simulink model "different_inverter_controls_BPS"  (R2024b)
settings: Solver=ode4  StartTime=0.0  StopTime=5  FixedStep=Ts  RelTol=1e-3
InitFcn:
  | %mode_of_operation=1;
  | %BESS_control_mode=1;
  | %Gen_Q_Control =1;
  | 
  | %Exciter_init;
  | 
  | %Exciter_init
  | Xq=0.474;
  | %%====================================================
  | % ST6C Exciter Parameters
  | 
  | KPA=30;
  | KIA=59.91;
  | KFF=1;
  | KM=1;
  | KLR=22.47;
  | KCL=1.04;
  | VAMAX=7.05;
  | VAMIN=-6.11;
  | VRMAX=7.05;
  | VRMIN=-6.11;
  | ILR=5.02;
  | KG=1;
  | TG=0.024;
  | TA=0.01;
  | VBMAX=999;
  | VMMAX=7.05;
  | VMMIN=-6.11;
  | KI=0;
  | Kp=1;
  | Kc=0;
  | Vt0=0;
  | VAAMAX=VAMAX;
  | %%========================================================
  | % UEL2C parameters
  | 
  | TUQ=.005;
  | TUP=0.050;
  | TUV=0.2;
  | TQREF=0;
  | Tadj=0;
  | K1=0;
  | K2=2;
  | VBIAS=1;
  | KFB=0;
  | TUL=0;
  | VUImax=1;
  | VUImin=-1;
  | VUELmax1=1;
  | VUELmax2=1;
  | VUELmin1=-1;
  | VUELmin2=-1;
  | KUF=0;
  | KUL=0.24;
  | KUI=0.001;
  | TU1=0;TU2=0;TU3=0;TU4=0;
  | KFIX=1;
  | VF=0;
  | VFB=0;
  | %%===========================================================
  | ... (+60 lines)
values from neighbouring files (symbols this model uses):
  inv1 = struct    [multiInverterParams.m]
  kp_sync = KQ_p/10    (= 0.04)    [multiInverterParams.m]
  Vdc = 1000    [multiInverterParams.m]
  Vpp = 480    [multiInverterParams.m]
undefined symbols (not defined in the file or in its folder): D1, Delta, DiscIntNeverNeededParam, Ion, Lithium, sigbuilder_block, sps
libraries: slpidlib x34, spsThreePhaseVIMeasurementLib x31, spsThreePhaseSeriesRLCBranchLib x23, spsabctodq0Lib x22, spsPower3phInstantaneousLib x22, spsThreePhaseTransformerTwoWindingsLib x16, spsSeriesRLCBranchLib x16, spsThreePhaseSeriesRLCLoadLib x14, simulink x12, spsPLL3phLib x11, spsGroundLib x9, powerlib_extras x8
(part 8 of 9)

== system different_inverter_controls_BPS/IBR-GFM PV Droop/IBR/Power Controller/P,Q Control /Integrator1 ==
  w : Inport
  Constant1 : Constant  Commented=on  Value=2*pi  SampleTime=Ts
  Constant2 : Constant  Value=2*pi  SampleTime=Ts_Control
  Constant3 : Constant  Commented=on  Value=2*pi  SampleTime=Ts
  Constant4 : Constant  Commented=on  Value=f  SampleTime=Ts_Control
  Constant5 : Constant  Commented=on  Value=0  SampleTime=Ts_Control
  Discrete-Time Integrator : DiscreteIntegrator  Commented=on  IntegratorMethod=Integration: Trapezoidal  SampleTime=Ts  ICPrevOutput=DiscIntNeverNeededParam  ICPrevScaledInput=DiscIntNeverNeededParam
  Discrete-Time Integrator1 : DiscreteIntegrator  ExternalReset=rising  InitialConditionSource=external  SampleTime=Ts_Control  ShowStatePort=on  ICPrevOutput=DiscIntNeverNeededParam  ICPrevScaledInput=DiscIntNeverNeededParam
  Divide : Product  Commented=on  Inputs=*/
  From : From  Commented=on  GotoTag=fsys
  Gain : Gain  Commented=on  Gain=2*pi*f
  Gain1 : Gain  Commented=on  Gain=2*pi*f  SaturateOnIntegerOverflow=on  OutDataTypeStr=Inherit: Same as input  ParamDataTypeStr=Inherit: Same as input
  Gain3 : Gain  Gain=2*pi*f
  Hit Crossing : HitCross  Commented=on  HitCrossingOffset=pi  HitCrossingDirection=falling  ShowOutputPort=off
  Initial : InitialCondition  Value=0
  Initial1 : InitialCondition  Commented=on  Value=0
  Integrator : Integrator  Commented=on  ExternalReset=rising  InitialConditionSource=external  InitialCondition=sps.Phase_Init*pi/180  LimitOutput=on  ShowStatePort=on
  Integrator2 : Integrator  Commented=on  ExternalReset=rising  InitialConditionSource=external  InitialCondition=sps.Phase_Init*pi/180  ShowStatePort=on
  Math Function : Math  Commented=on  Operator=mod  SignedPower=on
  Relational Operator : RelationalOperator  Operator=>  OutDataTypeStr=boolean  InputSameDT=off
  Relational Operator1 : RelationalOperator  Commented=on  Operator=>  OutDataTypeStr=boolean  InputSameDT=off
  Scope : Scope
  Scope1 : Scope  Commented=on
  Scope2 : Scope  Commented=on
  Scope3 : Scope  Commented=on
  Subtract : Sum  Inputs=+-
  Subtract1 : Sum  Commented=on  Inputs=+-
  Sum1 : Sum  Commented=on  Inputs=|++
  Sum2 : Sum  Commented=on  Inputs=|+-
  Theta : Outport
  wires:
  Gain3/1 -> Discrete-Time Integrator1/1
  w/1 -> Sum2/1, Gain3/1
  Gain1/1 -> Integrator/1
  Initial1/1 -> Integrator/3
  Relational Operator1/1 -> Integrator/2
  Integrator/State -> Subtract1/1, Relational Operator1/1
  Constant1/1 -> Subtract1/2, Relational Operator1/2
  Integrator/1 -> Scope3/1, Hit Crossing/1
  Subtract1/1 -> Initial1/1
  Relational Operator/1 -> Discrete-Time Integrator1/2
  Initial/1 -> Discrete-Time Integrator1/3
  Discrete-Time Integrator1/State -> Subtract/1, Relational Operator/1
  Constant2/1 -> Subtract/2, Relational Operator/2
  Subtract/1 -> Initial/1
  Discrete-Time Integrator1/1 -> Scope/1, Theta/1
  Gain/1 -> Discrete-Time Integrator/1
  Discrete-Time Integrator/1 -> Math Function/1
  Constant3/1 -> Math Function/2
  Math Function/1 -> Scope1/1
  Sum1/1 -> Gain/1  "W"
  Constant5/1 -> Sum2/2
  Sum2/1 -> Scope2/1, Sum1/1  "W"
  From/1 -> Divide/1
  Constant4/1 -> Divide/2
  Divide/1 -> Sum1/2

== system different_inverter_controls_BPS/IBR-GFM Synchro-inverter/Inverter/Inverter Control/Current Control/Current Regulator ==
  note: Id positive --> The converter generates active power ("Inverter mode") = Active Power P positive
  note: Iq positive --> The converter absorbs reactive power ("Inductive mode") = Reactive Power Q negative
  note: Sign Convention: Current going out of the converter = positive current
  note: Current Regulator
      | ================
  VdVq_meas : Inport  PortDimensions=2
  IdIq_meas : Inport  Port=2  PortDimensions=2
  IdIq_ref : Inport  Port=3  PortDimensions=2
  Add1 : Sum  Inputs=++-
  Add2 : Sum
  Add3 : Sum  Inputs=+++
  Demux : Demux  Outputs=2
  Demux1 : Demux  Outputs=2
  Lff : Gain  Gain=inv1.Lpu  SaturateOnIntegerOverflow=on  OutDataTypeStr=Inherit: Same as input  ParamDataTypeStr=Inherit: Same as input
  "Lff  " : Gain  Gain=inv1.Lpu  SaturateOnIntegerOverflow=on  OutDataTypeStr=Inherit: Same as input  ParamDataTypeStr=Inherit: Same as input
  Lff  1 : Gain  Commented=on  Gain=Ltot_pu  SaturateOnIntegerOverflow=on  OutDataTypeStr=Inherit: Same as input  ParamDataTypeStr=Inherit: Same as input
  Mux : Mux  Inputs=2
  PI : slpidlib/PID Controller  Controller=PI  Form=Parallel  TimeDomain=Discrete-time  UseExternalTs=off  SampleTime=Ts_Control  IntegratorMethod=Forward Euler  FilterMethod=Forward Euler  ControllerParametersSource=internal  P=Kp_Ireg/10  I=Ki_Ireg  D=0  UseFilter=on  N=100  TunerSelectOption=Transfer Function Based (PID Tuner App)  InitialConditionSource=internal  InitialConditionForIntegrator=0  InitialConditionForFilter=0  DifferentiatorICPrevScaledInput=0  ExternalReset=none  TrackingMode=off  Kt=1  LimitOutput=on  SatLimitsSource=internal  UpperSaturationLimit=1.5  LowerSaturationLimit=-1.5  LinearizeAsGain=off  AntiWindupMode=back-calculation  Kb=1  POutMin=[]  POutMax=[]  IOutMin=[]  IOutMax=[]  DOutMin=[]  DOutMax=[]  NOutMin=[]  NOutMax=[]  SumOutMin=[]  SumOutMax=[]  SaturationOutMin=[]  SaturationOutMax=[]  PParamMin=[]  PParamMax=[]  IParamMin=[]  IParamMax=[]  DParamMin=[]  DParamMax=[]  NParamMin=[]  NParamMax=[]  KbParamMin=[]  KbParamMax=[]  KtParamMin=[]  KtParamMax=[]  KbOutMin=[]  KbOutMax=[]  KtOutMin=[]  KtOutMax=[]  IntegratorOutMin=[]  IntegratorOutMax=[]  FilterOutMin=[]  FilterOutMax=[]  SumI1OutMin=[]  SumI1OutMax=[]  SumI2OutMin=[]  SumI2OutMax=[]  SumI3OutMin=[]  SumI3OutMax=[]  SumI4OutMin=[]  SumI4OutMax=[]  SumDOutMin=[]  SumDOutMax=[]  DifferentiatorOutMin=[]  DifferentiatorOutMax=[]  FilterDiffOutCoefMin=[]  FilterDiffOutCoefMax=[]  ReciprocalOutMin=[]  ReciprocalOutMax=[]  SumDenOutMin=[]  SumDenOutMax=[]  SumNumOutMin=[]  SumNumOutMax=[]  DivideOutMin=[]  DivideOutMax=[]  UdiffTsProdOutMin=[]  UdiffTsProdOutMax=[]  NTsProdOutMin=[]  NTsProdOutMax=[]  UintegralTsProdOutMin=[]  UintegralTsProdOutMax=[]  UngainTsProdOutMin=[]  UngainTsProdOutMax=[]  FilterDenConstantOutDataTypeStr=Inherit: Inherit via back propagation  FilterDenConstantOutMin=[]  FilterDenConstantOutMax=[]  PCopyOutDataTypeStr=Inherit: Inherit via back propagation  PCopyOutMin=[]  PCopyOutMax=[]  NCopyOutDataTypeStr=Inherit: Inherit via back propagation  NCopyOutMin=[]  NCopyOutMax=[]  IntegratorContinuousStateAttributes=''  IntegratorStateMustResolveToSignalObject=off  IntegratorRTWStateStorageClass=Auto  FilterContinuousStateAttributes=''  FilterStateMustResolveToSignalObject=off  FilterRTWStateStorageClass=Auto  ParallelPVariant=InternalParameters  IdealPVariant=Disabled  IVariant=InternalParameters  DVariant=Disabled  IntegratorVariant=Discrete  SatVariant=Enabled  AWVariant=BackCalculation  PCopyVariant=Disabled  TRVariant=Disabled  FdbkBlocksVariant=Forward  IdealPFdbkVariant=Disabled  SatFdbkVariant=Disabled  DerivativeFilterVariant=Disabled  NVariant=Disabled  NCopyVariant=Disabled_SignalSpec  FilterICVariant=Disabled  IntegratorICVariant=InternalICs  ExternalResetVariant=Disabled  TRSumVariant=Passthrough  SumFdbkVariant=Disabled  SumVariant=Sum_PI  TsampFilterVariant=InternalTs  TsampNgainVariant=Passthrough  TsampIntegralVariant=Passthrough  ExternalSaturationOutDataTypeStr=Inherit: Same as second input
  PI1 : slpidlib/PID Controller  Commented=on  Controller=PI  Form=Parallel  TimeDomain=Discrete-time  UseExternalTs=off  SampleTime=Ts_Control  IntegratorMethod=Forward Euler  FilterMethod=Forward Euler  ControllerParametersSource=internal  P=Kp_Ireg  I=Ki_Ireg  D=0  UseFilter=on  N=100  TunerSelectOption=Transfer Function Based (PID Tuner App)  InitialConditionSource=internal  InitialConditionForIntegrator=0  InitialConditionForFilter=0  DifferentiatorICPrevScaledInput=0  ExternalReset=none  TrackingMode=off  Kt=1  LimitOutput=on  SatLimitsSource=internal  UpperSaturationLimit=1.5  LowerSaturationLimit=-1.5  LinearizeAsGain=off  AntiWindupMode=clamping  Kb=1  POutMin=[]  POutMax=[]  IOutMin=[]  IOutMax=[]  DOutMin=[]  DOutMax=[]  NOutMin=[]  NOutMax=[]  SumOutMin=[]  SumOutMax=[]  SaturationOutMin=[]  SaturationOutMax=[]  PParamMin=[]  PParamMax=[]  IParamMin=[]  IParamMax=[]  DParamMin=[]  DParamMax=[]  NParamMin=[]  NParamMax=[]  KbParamMin=[]  KbParamMax=[]  KtParamMin=[]  KtParamMax=[]  KbOutMin=[]  KbOutMax=[]  KtOutMin=[]  KtOutMax=[]  IntegratorOutMin=[]  IntegratorOutMax=[]  FilterOutMin=[]  FilterOutMax=[]  SumI1OutMin=[]  SumI1OutMax=[]  SumI2OutMin=[]  SumI2OutMax=[]  SumI3OutMin=[]  SumI3OutMax=[]  SumI4OutMin=[]  SumI4OutMax=[]  SumDOutMin=[]  SumDOutMax=[]  DifferentiatorOutMin=[]  DifferentiatorOutMax=[]  FilterDiffOutCoefMin=[]  FilterDiffOutCoefMax=[]  ReciprocalOutMin=[]  ReciprocalOutMax=[]  SumDenOutMin=[]  SumDenOutMax=[]  SumNumOutMin=[]  SumNumOutMax=[]  DivideOutMin=[]  DivideOutMax=[]  UdiffTsProdOutMin=[]  UdiffTsProdOutMax=[]  NTsProdOutMin=[]  NTsProdOutMax=[]  UintegralTsProdOutMin=[]  UintegralTsProdOutMax=[]  UngainTsProdOutMin=[]  UngainTsProdOutMax=[]  FilterDenConstantOutDataTypeStr=Inherit: Inherit via back propagation  FilterDenConstantOutMin=[]  FilterDenConstantOutMax=[]  PCopyOutDataTypeStr=Inherit: Inherit via back propagation  PCopyOutMin=[]  PCopyOutMax=[]  NCopyOutDataTypeStr=Inherit: Inherit via back propagation  NCopyOutMin=[]  NCopyOutMax=[]  IntegratorContinuousStateAttributes=''  IntegratorStateMustResolveToSignalObject=off  IntegratorRTWStateStorageClass=Auto  FilterContinuousStateAttributes=''  FilterStateMustResolveToSignalObject=off  FilterRTWStateStorageClass=Auto  ParallelPVariant=InternalParameters  IdealPVariant=Disabled  IVariant=InternalParameters  DVariant=Disabled  IntegratorVariant=Discrete  SatVariant=Enabled  AWVariant=DiscClampingParallel  PCopyVariant=Disabled  TRVariant=Disabled  FdbkBlocksVariant=Forward  IdealPFdbkVariant=Disabled  SatFdbkVariant=Disabled  DerivativeFilterVariant=Disabled  NVariant=Disabled  NCopyVariant=Disabled_SignalSpec  FilterICVariant=Disabled  IntegratorICVariant=InternalICs  ExternalResetVariant=Disabled  TRSumVariant=Passthrough  SumFdbkVariant=Disabled  SumVariant=Sum_PI  TsampFilterVariant=InternalTs  TsampNgainVariant=Passthrough  TsampIntegralVariant=Passthrough  ExternalSaturationOutDataTypeStr=Inherit: Same as second input
  PI2 : slpidlib/PID Controller  Commented=on  Controller=PI  Form=Parallel  TimeDomain=Discrete-time  UseExternalTs=off  SampleTime=Ts_Control  IntegratorMethod=Forward Euler  FilterMethod=Forward Euler  ControllerParametersSource=internal  P=Kp_Ireg  I=Ki_Ireg  D=0  UseFilter=on  N=100  TunerSelectOption=Transfer Function Based (PID Tuner App)  InitialConditionSource=internal  InitialConditionForIntegrator=0  InitialConditionForFilter=0  DifferentiatorICPrevScaledInput=0  ExternalReset=none  TrackingMode=off  Kt=1  LimitOutput=on  SatLimitsSource=internal  UpperSaturationLimit=1.5  LowerSaturationLimit=-1.5  LinearizeAsGain=off  AntiWindupMode=back-calculation  Kb=1  POutMin=[]  POutMax=[]  IOutMin=[]  IOutMax=[]  DOutMin=[]  DOutMax=[]  NOutMin=[]  NOutMax=[]  SumOutMin=[]  SumOutMax=[]  SaturationOutMin=[]  SaturationOutMax=[]  PParamMin=[]  PParamMax=[]  IParamMin=[]  IParamMax=[]  DParamMin=[]  DParamMax=[]  NParamMin=[]  NParamMax=[]  KbParamMin=[]  KbParamMax=[]  KtParamMin=[]  KtParamMax=[]  KbOutMin=[]  KbOutMax=[]  KtOutMin=[]  KtOutMax=[]  IntegratorOutMin=[]  IntegratorOutMax=[]  FilterOutMin=[]  FilterOutMax=[]  SumI1OutMin=[]  SumI1OutMax=[]  SumI2OutMin=[]  SumI2OutMax=[]  SumI3OutMin=[]  SumI3OutMax=[]  SumI4OutMin=[]  SumI4OutMax=[]  SumDOutMin=[]  SumDOutMax=[]  DifferentiatorOutMin=[]  DifferentiatorOutMax=[]  FilterDiffOutCoefMin=[]  FilterDiffOutCoefMax=[]  ReciprocalOutMin=[]  ReciprocalOutMax=[]  SumDenOutMin=[]  SumDenOutMax=[]  SumNumOutMin=[]  SumNumOutMax=[]  DivideOutMin=[]  DivideOutMax=[]  UdiffTsProdOutMin=[]  UdiffTsProdOutMax=[]  NTsProdOutMin=[]  NTsProdOutMax=[]  UintegralTsProdOutMin=[]  UintegralTsProdOutMax=[]  UngainTsProdOutMin=[]  UngainTsProdOutMax=[]  FilterDenConstantOutDataTypeStr=Inherit: Inherit via back propagation  FilterDenConstantOutMin=[]  FilterDenConstantOutMax=[]  PCopyOutDataTypeStr=Inherit: Inherit via back propagation  PCopyOutMin=[]  PCopyOutMax=[]  NCopyOutDataTypeStr=Inherit: Inherit via back propagation  NCopyOutMin=[]  NCopyOutMax=[]  IntegratorContinuousStateAttributes=''  IntegratorStateMustResolveToSignalObject=off  IntegratorRTWStateStorageClass=Auto  FilterContinuousStateAttributes=''  FilterStateMustResolveToSignalObject=off  FilterRTWStateStorageClass=Auto  ParallelPVariant=InternalParameters  IdealPVariant=Disabled  IVariant=InternalParameters  DVariant=Disabled  IntegratorVariant=Discrete  SatVariant=Enabled  AWVariant=BackCalculation  PCopyVariant=Disabled  TRVariant=Disabled  FdbkBlocksVariant=Forward  IdealPFdbkVariant=Disabled  SatFdbkVariant=Disabled  DerivativeFilterVariant=Disabled  NVariant=Disabled  NCopyVariant=Disabled_SignalSpec  FilterICVariant=Disabled  IntegratorICVariant=InternalICs  ExternalResetVariant=Disabled  TRSumVariant=Passthrough  SumFdbkVariant=Disabled  SumVariant=Sum_PI  TsampFilterVariant=InternalTs  TsampNgainVariant=Passthrough  TsampIntegralVariant=Passthrough  ExternalSaturationOutDataTypeStr=Inherit: Same as second input
  Rff : Gain  Commented=on  Gain=inv1.R/inv1.Zb  SaturateOnIntegerOverflow=on  OutDataTypeStr=Inherit: Same as input  ParamDataTypeStr=Inherit: Same as input
  "Rff " : Gain  Commented=on  Gain=inv1.R/inv1.Zb  SaturateOnIntegerOverflow=on  OutDataTypeStr=Inherit: Same as input  ParamDataTypeStr=Inherit: Same as input
  Rff 1 : Gain  Commented=on  Gain=Rtot_pu  SaturateOnIntegerOverflow=on  OutDataTypeStr=Inherit: Same as input  ParamDataTypeStr=Inherit: Same as input
  Saturation : Saturate  UpperLimit=1.5  LowerLimit=-1.5
  Scope : Scope  NumInputPorts=2
  Scope1 : Scope
  Sum : Sum  Inputs=|-+
  VdVq_conv : Outport  VectorParamsAs1DForOutWhenUnconnected=off
  wires:
  Add3/1 -> Mux/2
  Demux/2 -> Add3/1
  Add1/1 -> Mux/1  "Feedforward"
  Lff/1 -> Add3/3
  Rff/1 -> Add3/2
  Demux1/2 -> Rff/1, "Lff  "/1
  "Lff  "/1 -> Add1/3
  Demux1/1 -> Lff/1, "Rff "/1
  "Rff "/1 -> Add1/2
  Demux/1 -> Add1/1
  VdVq_meas/1 -> Demux/1
  Saturation/1 -> VdVq_conv/1, Scope1/1
  Add2/1 -> Saturation/1
  IdIq_meas/1 -> Sum/1, Demux1/1
  IdIq_ref/1 -> Sum/2
  Sum/1 -> PI/1, Scope/1
  PI/1 -> Add2/1, Scope/2  "PI"
  Mux/1 -> Add2/2

== system different_inverter_controls_BPS/IBR-GFM Synchro-inverter/Inverter/Inverter Control/Current Control/Uabc_ref Generation max (m) = 1 ==
  note: Uref Generation
      | ==============
  note: (Correction for delay of Ts_Control)
  note: (Correction for transformer
      |  D1 connection)
  wt : Inport
  VdVq_conv : Inport  Port=2
  Add1 : Sum  Inputs=++++
  Add2 : Sum
  Complex to Magnitude-Angle : ComplexToMagnitudeAngle
  Constant : Constant  Commented=on  Value=-pi/6
  Constant1 : Constant  Commented=on  Value=Vnom_dc
  Constant2 : Constant  Value="[ 0  -2*pi/3  2*pi/3  ]"
  Constant3 : Constant  Commented=on  Value=Vnom_sec*sqrt(2)/sqrt(3)
  Constant4 : Constant  Value=Ts_Control*Fnom*(2*pi)
  Constant5 : Constant  Value=Vdc
  Constant6 : Constant  Value=Vpp*sqrt(2)/sqrt(3)
  Demux1 : Demux  Outputs=2
  Gain1 : Gain  Gain=1/2
  Product : Product  Inputs=*/  RndMeth=Zero
  Product1 : Product  Inputs=*/  RndMeth=Zero
  Product2 : Product  Inputs=**  RndMeth=Zero
  Real-Imag to Complex : RealImagToComplex
  Trigonometric Function : Trigonometry
  Uabc_ref : Outport  VectorParamsAs1DForOutWhenUnconnected=off
  wires:
  Product/1 -> Product1/2
  Constant4/1 -> Add1/4
  wt/1 -> Add1/1
  Product2/1 -> Uabc_ref/1
  Trigonometric Function/1 -> Product2/2
  Complex to Magnitude-Angle/1 -> Product2/1
  Add2/1 -> Trigonometric Function/1
  Add1/1 -> Add2/2
  Complex to Magnitude-Angle/2 -> Add2/1
  Constant6/1 -> Product/2
  Constant/1 -> Add1/3
  Constant2/1 -> Add1/2
  Demux1/2 -> Real-Imag to Complex/2
  Demux1/1 -> Real-Imag to Complex/1
  Real-Imag to Complex/1 -> Complex to Magnitude-Angle/1
  Gain1/1 -> Product/1
  Product1/1 -> Demux1/1
  VdVq_conv/1 -> Product1/1
  Constant5/1 -> Gain1/1

== system different_inverter_controls_BPS/IBR-GFM Synchro-inverter/Inverter/Inverter Control/current limiter/P priority limit ==
  idiqP : Inport
  Demux4 : Demux  Outputs=2
  IqLimit : Subsystem
  Mux4 : Mux  Inputs=2
  Rtot_pu1 : Gain  Gain=-1  SaturateOnIntegerOverflow=on  OutDataTypeStr=Inherit: Same as input  ParamDataTypeStr=Inherit: Same as input
  Saturation : Saturate  UpperLimit=limMax  LowerLimit=0
  Saturation Dynamic : simulink/Discontinuities/Saturation Dynamic  OutMin=[]  OutMax=[limMax]  OutDataTypeStr=Inherit: Same as second input  OutDataType=fixdt(1, 16)  OutScaling=2^-10  DoSatur=off
  idiqPRefL : Outport
  wires:
  Saturation Dynamic/1 -> Mux4/2
  idiqP/1 -> Demux4/1
  Demux4/2 -> Saturation Dynamic/2
  Mux4/1 -> idiqPRefL/1
  Demux4/1 -> Saturation/1
  Saturation/1 -> IqLimit/1(In1), Mux4/1
  Rtot_pu1/1 -> Saturation Dynamic/3
  IqLimit/1(Out2) -> Rtot_pu1/1, Saturation Dynamic/1

== system different_inverter_controls_BPS/IBR-GFM Synchro-inverter/Inverter/Inverter Control/current limiter/Q priority limit ==
  idiqP : Inport
  V_inv_mag : Inport  Port=2
  Demux4 : Demux  Outputs=2
  Iq condition : Switch  Threshold=0.9  SaturateOnIntegerOverflow=off  InputSameDT=off
  IqLimit : Subsystem
  Mux4 : Mux  Inputs=2
  Rtot_pu1 : Gain  Gain=-1  SaturateOnIntegerOverflow=on  OutDataTypeStr=Inherit: Same as input  ParamDataTypeStr=Inherit: Same as input
  Saturation : Saturate  UpperLimit=limMax  LowerLimit=limMin
  Saturation Dynamic : simulink/Discontinuities/Saturation Dynamic  OutMin=[]  OutMax=[]  OutDataTypeStr=Inherit: Same as second input  OutDataType=fixdt(1, 16)  OutScaling=2^-10  DoSatur=off
  Saturation1 : Saturate  UpperLimit=0  LowerLimit=limMin
  Scope : Scope
  idiqPRefL : Outport
  wires:
  Iq condition/1 -> Mux4/2, IqLimit/1(In1)
  V_inv_mag/1 -> Iq condition/2
  Saturation/1 -> Iq condition/1
  idiqP/1 -> Demux4/1
  Mux4/1 -> idiqPRefL/1
  Rtot_pu1/1 -> Saturation Dynamic/3
  Saturation Dynamic/1 -> Mux4/1
  Demux4/1 -> Saturation Dynamic/2
  IqLimit/1(Out2) -> Rtot_pu1/1, Saturation Dynamic/1
  Saturation1/1 -> Iq condition/3
  Demux4/2 -> Saturation/1, Saturation1/1

== system different_inverter_controls_BPS/IBR-GFM Synchro-inverter/Inverter/Inverter Control/current limiter/Subsystem3 ==
  In1 : Inport
  Demux2 : Demux  Outputs=2
  Math Function : Math  Operator=square  SignedPower=on
  Saturation : Saturate  UpperLimit=limMax  LowerLimit=limMin
  Scope : Scope  NumInputPorts=2
  Sqrt1 : Sqrt
  Subtract : Sum
  Out1 : Outport
  Out2 : Outport  Port=2
  wires:
  Demux2/2 -> Subtract/2
  Demux2/1 -> Subtract/1
  Math Function/1 -> Demux2/1
  In1/1 -> Scope/2, Math Function/1
  Subtract/1 -> Sqrt1/1  "Ipos2"
  Sqrt1/1 -> Saturation/1, Scope/1, Out2/1
  Saturation/1 -> Out1/1

== system different_inverter_controls_BPS/IBR-GFM Synchro-inverter/Inverter/Inverter Control/current limiter/Subsystem4 ==
  In1 : Inport
  In2 : Inport  Port=2
  Demux4 : Demux  Outputs=2
  Mux4 : Mux  Inputs=2
  Switch1 : Switch  Threshold=limMax  SaturateOnIntegerOverflow=off  InputSameDT=off
  Unit Delay2 : UnitDelay  InitialCondition=1  SampleTime=Ts_Control  HasFrameUpgradeWarning=on
  dummy limit : Saturate  UpperLimit=limMax  LowerLimit=limMin
  Out1 : Outport
  wires:
  Switch1/1 -> Out1/1, Mux4/1, Unit Delay2/1
  Unit Delay2/1 -> Switch1/1
  In1/1 -> Switch1/2
  In2/1 -> Switch1/3, Demux4/1
  Demux4/2 -> dummy limit/1
  dummy limit/1 -> Mux4/2

== system different_inverter_controls_BPS/IBR-GFM Synchro-inverter/Inverter/Inverter Control/current limiter/Subsystem9 ==
  In1 : Inport
  In2 : Inport  Port=2
  Divide : Product  Inputs=*/
  Gain1 : Gain  Gain=limMax
  Saturation : Saturate  UpperLimit=limMax  LowerLimit=limMin
  Switch1 : Switch  Threshold=limMax  SaturateOnIntegerOverflow=off  InputSameDT=off
  idiqPRefL : Outport
  wires:
  In1/1 -> Divide/2, Switch1/2
  In2/1 -> Divide/1, Switch1/3
  Divide/1 -> Gain1/1
  Gain1/1 -> Switch1/1
  Switch1/1 -> Saturation/1
  Saturation/1 -> idiqPRefL/1

== system different_inverter_controls_BPS/IBR-GFM Synchro-inverter/Inverter/Power Controller/P,Q Control /Integrator ==
  w : Inport
  Constant1 : Constant  Commented=on  Value=2*pi  SampleTime=Ts
  Constant2 : Constant  Value=2*pi  SampleTime=Ts_Control
  Constant3 : Constant  Commented=on  Value=2*pi  SampleTime=Ts
  Constant4 : Constant  Commented=on  Value=f  SampleTime=Ts_Control
  Constant5 : Constant  Commented=on  Value=0  SampleTime=Ts_Control
  Discrete-Time Integrator : DiscreteIntegrator  Commented=on  IntegratorMethod=Integration: Trapezoidal  SampleTime=Ts  ICPrevOutput=DiscIntNeverNeededParam  ICPrevScaledInput=DiscIntNeverNeededParam
  Discrete-Time Integrator1 : DiscreteIntegrator  ExternalReset=rising  InitialConditionSource=external  SampleTime=Ts_Control  ShowStatePort=on  ICPrevOutput=DiscIntNeverNeededParam  ICPrevScaledInput=DiscIntNeverNeededParam
  Divide : Product  Commented=on  Inputs=*/
  From : From  Commented=on  GotoTag=fsys
  Gain : Gain  Commented=on  Gain=2*pi*f
  Gain1 : Gain  Commented=on  Gain=2*pi*f  SaturateOnIntegerOverflow=on  OutDataTypeStr=Inherit: Same as input  ParamDataTypeStr=Inherit: Same as input
  Gain3 : Gain  Gain=2*pi*f
  Hit Crossing : HitCross  Commented=on  HitCrossingOffset=pi  HitCrossingDirection=falling  ShowOutputPort=off
  Initial : InitialCondition  Value=0
  Initial1 : InitialCondition  Commented=on  Value=0
  Integrator : Integrator  Commented=on  ExternalReset=rising  InitialConditionSource=external  InitialCondition=sps.Phase_Init*pi/180  LimitOutput=on  ShowStatePort=on
  Integrator2 : Integrator  Commented=on  ExternalReset=rising  InitialConditionSource=external  InitialCondition=sps.Phase_Init*pi/180  ShowStatePort=on
  Math Function : Math  Commented=on  Operator=mod  SignedPower=on
  Relational Operator : RelationalOperator  Operator=>  OutDataTypeStr=boolean  InputSameDT=off
  Relational Operator1 : RelationalOperator  Commented=on  Operator=>  OutDataTypeStr=boolean  InputSameDT=off
  Scope : Scope
  Scope1 : Scope  Commented=on
  Scope2 : Scope  Commented=on
  Scope3 : Scope  Commented=on
  Subtract : Sum  Inputs=+-
  Subtract1 : Sum  Commented=on  Inputs=+-
  Sum1 : Sum  Commented=on  Inputs=|++
  Sum2 : Sum  Commented=on  Inputs=|+-
  Theta : Outport
  wires:
  Gain3/1 -> Discrete-Time Integrator1/1
  w/1 -> Sum2/1, Gain3/1
  Gain1/1 -> Integrator/1
  Initial1/1 -> Integrator/3
  Relational Operator1/1 -> Integrator/2
  Integrator/State -> Subtract1/1, Relational Operator1/1
  Constant1/1 -> Subtract1/2, Relational Operator1/2
  Integrator/1 -> Scope3/1, Hit Crossing/1
  Subtract1/1 -> Initial1/1
  Relational Operator/1 -> Discrete-Time Integrator1/2
  Initial/1 -> Discrete-Time Integrator1/3
  Discrete-Time Integrator1/State -> Subtract/1, Relational Operator/1
  Constant2/1 -> Subtract/2, Relational Operator/2
  Subtract/1 -> Initial/1
  Discrete-Time Integrator1/1 -> Scope/1, Theta/1
  Gain/1 -> Discrete-Time Integrator/1
  Discrete-Time Integrator/1 -> Math Function/1
  Constant3/1 -> Math Function/2
  Math Function/1 -> Scope1/1
  Sum1/1 -> Gain/1  "W"
  Constant5/1 -> Sum2/2
  Sum2/1 -> Scope2/1, Sum1/1  "W"
  From/1 -> Divide/1
  Constant4/1 -> Divide/2
  Divide/1 -> Sum1/2

== system different_inverter_controls_BPS/IBR-GFM Synchro-inverter/Inverter/Power Controller/P,Q Control /Integrator1 ==
  w : Inport
  Constant1 : Constant  Commented=on  Value=2*pi  SampleTime=Ts
  Constant2 : Constant  Value=2*pi  SampleTime=Ts_Control
  Constant3 : Constant  Commented=on  Value=2*pi  SampleTime=Ts
  Constant4 : Constant  Commented=on  Value=f  SampleTime=Ts_Control
  Constant5 : Constant  Commented=on  Value=0  SampleTime=Ts_Control
  Discrete-Time Integrator : DiscreteIntegrator  Commented=on  IntegratorMethod=Integration: Trapezoidal  SampleTime=Ts  ICPrevOutput=DiscIntNeverNeededParam  ICPrevScaledInput=DiscIntNeverNeededParam
  Discrete-Time Integrator1 : DiscreteIntegrator  ExternalReset=rising  InitialConditionSource=external  SampleTime=Ts_Control  ShowStatePort=on  ICPrevOutput=DiscIntNeverNeededParam  ICPrevScaledInput=DiscIntNeverNeededParam
  Divide : Product  Commented=on  Inputs=*/
  From : From  Commented=on  GotoTag=fsys
  Gain : Gain  Commented=on  Gain=2*pi*f
  Gain1 : Gain  Commented=on  Gain=2*pi*f  SaturateOnIntegerOverflow=on  OutDataTypeStr=Inherit: Same as input  ParamDataTypeStr=Inherit: Same as input
  Gain3 : Gain  Gain=2*pi*f
  Hit Crossing : HitCross  Commented=on  HitCrossingOffset=pi  HitCrossingDirection=falling  ShowOutputPort=off
  Initial : InitialCondition  Value=0
  Initial1 : InitialCondition  Commented=on  Value=0
  Integrator : Integrator  Commented=on  ExternalReset=rising  InitialConditionSource=external  InitialCondition=sps.Phase_Init*pi/180  LimitOutput=on  ShowStatePort=on
  Integrator2 : Integrator  Commented=on  ExternalReset=rising  InitialConditionSource=external  InitialCondition=sps.Phase_Init*pi/180  ShowStatePort=on
  Math Function : Math  Commented=on  Operator=mod  SignedPower=on
  Relational Operator : RelationalOperator  Operator=>  OutDataTypeStr=boolean  InputSameDT=off
  Relational Operator1 : RelationalOperator  Commented=on  Operator=>  OutDataTypeStr=boolean  InputSameDT=off
  Scope : Scope
  Scope1 : Scope  Commented=on
  Scope2 : Scope  Commented=on
  Scope3 : Scope  Commented=on
  Subtract : Sum  Inputs=+-
  Subtract1 : Sum  Commented=on  Inputs=+-
  Sum1 : Sum  Commented=on  Inputs=|++
  Sum2 : Sum  Commented=on  Inputs=|+-
  Theta : Outport
  wires:
  Divide/1 -> Sum1/2
  Constant4/1 -> Divide/2
  From/1 -> Divide/1
  Sum2/1 -> Sum1/1, Scope2/1  "W"
  Constant5/1 -> Sum2/2
  Sum1/1 -> Gain/1  "W"
  Math Function/1 -> Scope1/1
  Constant3/1 -> Math Function/2
  Discrete-Time Integrator/1 -> Math Function/1
  Gain/1 -> Discrete-Time Integrator/1
  Discrete-Time Integrator1/1 -> Theta/1, Scope/1
  Subtract/1 -> Initial/1
  Constant2/1 -> Relational Operator/2, Subtract/2
  Discrete-Time Integrator1/State -> Relational Operator/1, Subtract/1
  Initial/1 -> Discrete-Time Integrator1/3
  Relational Operator/1 -> Discrete-Time Integrator1/2
  Subtract1/1 -> Initial1/1
  Integrator/1 -> Hit Crossing/1, Scope3/1
  Constant1/1 -> Relational Operator1/2, Subtract1/2
  Integrator/State -> Relational Operator1/1, Subtract1/1
  Relational Operator1/1 -> Integrator/2
  Initial1/1 -> Integrator/3
  Gain1/1 -> Integrator/1
  w/1 -> Gain3/1, Sum2/1
  Gain3/1 -> Discrete-Time Integrator1/1

== system different_inverter_controls_BPS/IBR-GFM Power Synchronization/Inverter/Inverter Control/Current Control/Current Regulator ==
  note: Id positive --> The converter generates active power ("Inverter mode") = Active Power P positive
  note: Iq positive --> The converter absorbs reactive power ("Inductive mode") = Reactive Power Q negative
  note: Sign Convention: Current going out of the converter = positive current
  note: Current Regulator
      | ================
  VdVq_meas : Inport  PortDimensions=2
  IdIq_meas : Inport  Port=2  PortDimensions=2
  IdIq_ref : Inport  Port=3  PortDimensions=2
  Add1 : Sum  Inputs=++-
  Add2 : Sum
  Add3 : Sum  Inputs=+++
  Demux : Demux  Outputs=2
  Demux1 : Demux  Outputs=2
  Lff : Gain  Gain=inv1.Lpu  SaturateOnIntegerOverflow=on  OutDataTypeStr=Inherit: Same as input  ParamDataTypeStr=Inherit: Same as input
  "Lff  " : Gain  Gain=inv1.Lpu  SaturateOnIntegerOverflow=on  OutDataTypeStr=Inherit: Same as input  ParamDataTypeStr=Inherit: Same as input
  Lff  1 : Gain  Commented=on  Gain=Ltot_pu  SaturateOnIntegerOverflow=on  OutDataTypeStr=Inherit: Same as input  ParamDataTypeStr=Inherit: Same as input
  Mux : Mux  Inputs=2
  PI : slpidlib/PID Controller  Controller=PI  Form=Parallel  TimeDomain=Discrete-time  UseExternalTs=off  SampleTime=Ts_Control  IntegratorMethod=Forward Euler  FilterMethod=Forward Euler  ControllerParametersSource=internal  P=Kp_Ireg/10  I=Ki_Ireg  D=0  UseFilter=on  N=100  TunerSelectOption=Transfer Function Based (PID Tuner App)  InitialConditionSource=internal  InitialConditionForIntegrator=0  InitialConditionForFilter=0  DifferentiatorICPrevScaledInput=0  ExternalReset=none  TrackingMode=off  Kt=1  LimitOutput=on  SatLimitsSource=internal  UpperSaturationLimit=1.5  LowerSaturationLimit=-1.5  LinearizeAsGain=off  AntiWindupMode=back-calculation  Kb=1  POutMin=[]  POutMax=[]  IOutMin=[]  IOutMax=[]  DOutMin=[]  DOutMax=[]  NOutMin=[]  NOutMax=[]  SumOutMin=[]  SumOutMax=[]  SaturationOutMin=[]  SaturationOutMax=[]  PParamMin=[]  PParamMax=[]  IParamMin=[]  IParamMax=[]  DParamMin=[]  DParamMax=[]  NParamMin=[]  NParamMax=[]  KbParamMin=[]  KbParamMax=[]  KtParamMin=[]  KtParamMax=[]  KbOutMin=[]  KbOutMax=[]  KtOutMin=[]  KtOutMax=[]  IntegratorOutMin=[]  IntegratorOutMax=[]  FilterOutMin=[]  FilterOutMax=[]  SumI1OutMin=[]  SumI1OutMax=[]  SumI2OutMin=[]  SumI2OutMax=[]  SumI3OutMin=[]  SumI3OutMax=[]  SumI4OutMin=[]  SumI4OutMax=[]  SumDOutMin=[]  SumDOutMax=[]  DifferentiatorOutMin=[]  DifferentiatorOutMax=[]  FilterDiffOutCoefMin=[]  FilterDiffOutCoefMax=[]  ReciprocalOutMin=[]  ReciprocalOutMax=[]  SumDenOutMin=[]  SumDenOutMax=[]  SumNumOutMin=[]  SumNumOutMax=[]  DivideOutMin=[]  DivideOutMax=[]  UdiffTsProdOutMin=[]  UdiffTsProdOutMax=[]  NTsProdOutMin=[]  NTsProdOutMax=[]  UintegralTsProdOutMin=[]  UintegralTsProdOutMax=[]  UngainTsProdOutMin=[]  UngainTsProdOutMax=[]  FilterDenConstantOutDataTypeStr=Inherit: Inherit via back propagation  FilterDenConstantOutMin=[]  FilterDenConstantOutMax=[]  PCopyOutDataTypeStr=Inherit: Inherit via back propagation  PCopyOutMin=[]  PCopyOutMax=[]  NCopyOutDataTypeStr=Inherit: Inherit via back propagation  NCopyOutMin=[]  NCopyOutMax=[]  IntegratorContinuousStateAttributes=''  IntegratorStateMustResolveToSignalObject=off  IntegratorRTWStateStorageClass=Auto  FilterContinuousStateAttributes=''  FilterStateMustResolveToSignalObject=off  FilterRTWStateStorageClass=Auto  ParallelPVariant=InternalParameters  IdealPVariant=Disabled  IVariant=InternalParameters  DVariant=Disabled  IntegratorVariant=Discrete  SatVariant=Enabled  AWVariant=BackCalculation  PCopyVariant=Disabled  TRVariant=Disabled  FdbkBlocksVariant=Forward  IdealPFdbkVariant=Disabled  SatFdbkVariant=Disabled  DerivativeFilterVariant=Disabled  NVariant=Disabled  NCopyVariant=Disabled_SignalSpec  FilterICVariant=Disabled  IntegratorICVariant=InternalICs  ExternalResetVariant=Disabled  TRSumVariant=Passthrough  SumFdbkVariant=Disabled  SumVariant=Sum_PI  TsampFilterVariant=InternalTs  TsampNgainVariant=Passthrough  TsampIntegralVariant=Passthrough  ExternalSaturationOutDataTypeStr=Inherit: Same as second input
  PI1 : slpidlib/PID Controller  Commented=on  Controller=PI  Form=Parallel  TimeDomain=Discrete-time  UseExternalTs=off  SampleTime=Ts_Control  IntegratorMethod=Forward Euler  FilterMethod=Forward Euler  ControllerParametersSource=internal  P=Kp_Ireg  I=Ki_Ireg  D=0  UseFilter=on  N=100  TunerSelectOption=Transfer Function Based (PID Tuner App)  InitialConditionSource=internal  InitialConditionForIntegrator=0  InitialConditionForFilter=0  DifferentiatorICPrevScaledInput=0  ExternalReset=none  TrackingMode=off  Kt=1  LimitOutput=on  SatLimitsSource=internal  UpperSaturationLimit=1.5  LowerSaturationLimit=-1.5  LinearizeAsGain=off  AntiWindupMode=clamping  Kb=1  POutMin=[]  POutMax=[]  IOutMin=[]  IOutMax=[]  DOutMin=[]  DOutMax=[]  NOutMin=[]  NOutMax=[]  SumOutMin=[]  SumOutMax=[]  SaturationOutMin=[]  SaturationOutMax=[]  PParamMin=[]  PParamMax=[]  IParamMin=[]  IParamMax=[]  DParamMin=[]  DParamMax=[]  NParamMin=[]  NParamMax=[]  KbParamMin=[]  KbParamMax=[]  KtParamMin=[]  KtParamMax=[]  KbOutMin=[]  KbOutMax=[]  KtOutMin=[]  KtOutMax=[]  IntegratorOutMin=[]  IntegratorOutMax=[]  FilterOutMin=[]  FilterOutMax=[]  SumI1OutMin=[]  SumI1OutMax=[]  SumI2OutMin=[]  SumI2OutMax=[]  SumI3OutMin=[]  SumI3OutMax=[]  SumI4OutMin=[]  SumI4OutMax=[]  SumDOutMin=[]  SumDOutMax=[]  DifferentiatorOutMin=[]  DifferentiatorOutMax=[]  FilterDiffOutCoefMin=[]  FilterDiffOutCoefMax=[]  ReciprocalOutMin=[]  ReciprocalOutMax=[]  SumDenOutMin=[]  SumDenOutMax=[]  SumNumOutMin=[]  SumNumOutMax=[]  DivideOutMin=[]  DivideOutMax=[]  UdiffTsProdOutMin=[]  UdiffTsProdOutMax=[]  NTsProdOutMin=[]  NTsProdOutMax=[]  UintegralTsProdOutMin=[]  UintegralTsProdOutMax=[]  UngainTsProdOutMin=[]  UngainTsProdOutMax=[]  FilterDenConstantOutDataTypeStr=Inherit: Inherit via back propagation  FilterDenConstantOutMin=[]  FilterDenConstantOutMax=[]  PCopyOutDataTypeStr=Inherit: Inherit via back propagation  PCopyOutMin=[]  PCopyOutMax=[]  NCopyOutDataTypeStr=Inherit: Inherit via back propagation  NCopyOutMin=[]  NCopyOutMax=[]  IntegratorContinuousStateAttributes=''  IntegratorStateMustResolveToSignalObject=off  IntegratorRTWStateStorageClass=Auto  FilterContinuousStateAttributes=''  FilterStateMustResolveToSignalObject=off  FilterRTWStateStorageClass=Auto  ParallelPVariant=InternalParameters  IdealPVariant=Disabled  IVariant=InternalParameters  DVariant=Disabled  IntegratorVariant=Discrete  SatVariant=Enabled  AWVariant=DiscClampingParallel  PCopyVariant=Disabled  TRVariant=Disabled  FdbkBlocksVariant=Forward  IdealPFdbkVariant=Disabled  SatFdbkVariant=Disabled  DerivativeFilterVariant=Disabled  NVariant=Disabled  NCopyVariant=Disabled_SignalSpec  FilterICVariant=Disabled  IntegratorICVariant=InternalICs  ExternalResetVariant=Disabled  TRSumVariant=Passthrough  SumFdbkVariant=Disabled  SumVariant=Sum_PI  TsampFilterVariant=InternalTs  TsampNgainVariant=Passthrough  TsampIntegralVariant=Passthrough  ExternalSaturationOutDataTypeStr=Inherit: Same as second input
  PI2 : slpidlib/PID Controller  Commented=on  Controller=PI  Form=Parallel  TimeDomain=Discrete-time  UseExternalTs=off  SampleTime=Ts_Control  IntegratorMethod=Forward Euler  FilterMethod=Forward Euler  ControllerParametersSource=internal  P=Kp_Ireg  I=Ki_Ireg  D=0  UseFilter=on  N=100  TunerSelectOption=Transfer Function Based (PID Tuner App)  InitialConditionSource=internal  InitialConditionForIntegrator=0  InitialConditionForFilter=0  DifferentiatorICPrevScaledInput=0  ExternalReset=none  TrackingMode=off  Kt=1  LimitOutput=on  SatLimitsSource=internal  UpperSaturationLimit=1.5  LowerSaturationLimit=-1.5  LinearizeAsGain=off  AntiWindupMode=back-calculation  Kb=1  POutMin=[]  POutMax=[]  IOutMin=[]  IOutMax=[]  DOutMin=[]  DOutMax=[]  NOutMin=[]  NOutMax=[]  SumOutMin=[]  SumOutMax=[]  SaturationOutMin=[]  SaturationOutMax=[]  PParamMin=[]  PParamMax=[]  IParamMin=[]  IParamMax=[]  DParamMin=[]  DParamMax=[]  NParamMin=[]  NParamMax=[]  KbParamMin=[]  KbParamMax=[]  KtParamMin=[]  KtParamMax=[]  KbOutMin=[]  KbOutMax=[]  KtOutMin=[]  KtOutMax=[]  IntegratorOutMin=[]  IntegratorOutMax=[]  FilterOutMin=[]  FilterOutMax=[]  SumI1OutMin=[]  SumI1OutMax=[]  SumI2OutMin=[]  SumI2OutMax=[]  SumI3OutMin=[]  SumI3OutMax=[]  SumI4OutMin=[]  SumI4OutMax=[]  SumDOutMin=[]  SumDOutMax=[]  DifferentiatorOutMin=[]  DifferentiatorOutMax=[]  FilterDiffOutCoefMin=[]  FilterDiffOutCoefMax=[]  ReciprocalOutMin=[]  ReciprocalOutMax=[]  SumDenOutMin=[]  SumDenOutMax=[]  SumNumOutMin=[]  SumNumOutMax=[]  DivideOutMin=[]  DivideOutMax=[]  UdiffTsProdOutMin=[]  UdiffTsProdOutMax=[]  NTsProdOutMin=[]  NTsProdOutMax=[]  UintegralTsProdOutMin=[]  UintegralTsProdOutMax=[]  UngainTsProdOutMin=[]  UngainTsProdOutMax=[]  FilterDenConstantOutDataTypeStr=Inherit: Inherit via back propagation  FilterDenConstantOutMin=[]  FilterDenConstantOutMax=[]  PCopyOutDataTypeStr=Inherit: Inherit via back propagation  PCopyOutMin=[]  PCopyOutMax=[]  NCopyOutDataTypeStr=Inherit: Inherit via back propagation  NCopyOutMin=[]  NCopyOutMax=[]  IntegratorContinuousStateAttributes=''  IntegratorStateMustResolveToSignalObject=off  IntegratorRTWStateStorageClass=Auto  FilterContinuousStateAttributes=''  FilterStateMustResolveToSignalObject=off  FilterRTWStateStorageClass=Auto  ParallelPVariant=InternalParameters  IdealPVariant=Disabled  IVariant=InternalParameters  DVariant=Disabled  IntegratorVariant=Discrete  SatVariant=Enabled  AWVariant=BackCalculation  PCopyVariant=Disabled  TRVariant=Disabled  FdbkBlocksVariant=Forward  IdealPFdbkVariant=Disabled  SatFdbkVariant=Disabled  DerivativeFilterVariant=Disabled  NVariant=Disabled  NCopyVariant=Disabled_SignalSpec  FilterICVariant=Disabled  IntegratorICVariant=InternalICs  ExternalResetVariant=Disabled  TRSumVariant=Passthrough  SumFdbkVariant=Disabled  SumVariant=Sum_PI  TsampFilterVariant=InternalTs  TsampNgainVariant=Passthrough  TsampIntegralVariant=Passthrough  ExternalSaturationOutDataTypeStr=Inherit: Same as second input
  Rff : Gain  Commented=on  Gain=inv1.R/inv1.Zb  SaturateOnIntegerOverflow=on  OutDataTypeStr=Inherit: Same as input  ParamDataTypeStr=Inherit: Same as input
  "Rff " : Gain  Commented=on  Gain=inv1.R/inv1.Zb  SaturateOnIntegerOverflow=on  OutDataTypeStr=Inherit: Same as input  ParamDataTypeStr=Inherit: Same as input
  Rff 1 : Gain  Commented=on  Gain=Rtot_pu  SaturateOnIntegerOverflow=on  OutDataTypeStr=Inherit: Same as input  ParamDataTypeStr=Inherit: Same as input
  Saturation : Saturate  UpperLimit=1.5  LowerLimit=-1.5
  Scope : Scope  NumInputPorts=2
  Scope1 : Scope
  Sum : Sum  Inputs=|-+
  VdVq_conv : Outport  VectorParamsAs1DForOutWhenUnconnected=off
  wires:
  Add3/1 -> Mux/2
  Demux/2 -> Add3/1
  Add1/1 -> Mux/1  "Feedforward"
  Lff/1 -> Add3/3
  Rff/1 -> Add3/2
  Demux1/2 -> Rff/1, "Lff  "/1
  "Lff  "/1 -> Add1/3
  Demux1/1 -> Lff/1, "Rff "/1
  "Rff "/1 -> Add1/2
  Demux/1 -> Add1/1
  VdVq_meas/1 -> Demux/1
  Saturation/1 -> VdVq_conv/1, Scope1/1
  Add2/1 -> Saturation/1
  IdIq_meas/1 -> Sum/1, Demux1/1
  IdIq_ref/1 -> Sum/2
  Sum/1 -> PI/1, Scope/1
  PI/1 -> Add2/1, Scope/2  "PI"
  Mux/1 -> Add2/2

== system different_inverter_controls_BPS/IBR-GFM Power Synchronization/Inverter/Inverter Control/Current Control/Uabc_ref Generation max (m) = 1 ==
  note: Uref Generation
      | ==============
  note: (Correction for delay of Ts_Control)
  note: (Correction for transformer
      |  D1 connection)
  wt : Inport
  VdVq_conv : Inport  Port=2
  Add1 : Sum  Inputs=++++
  Add2 : Sum
  Complex to Magnitude-Angle : ComplexToMagnitudeAngle
  Constant : Constant  Commented=on  Value=-pi/6
  Constant1 : Constant  Commented=on  Value=Vnom_dc
  Constant2 : Constant  Value="[ 0  -2*pi/3  2*pi/3  ]"
  Constant3 : Constant  Commented=on  Value=Vnom_sec*sqrt(2)/sqrt(3)
  Constant4 : Constant  Value=Ts_Control*Fnom*(2*pi)
  Constant5 : Constant  Value=Vdc
  Constant6 : Constant  Value=Vpp*sqrt(2)/sqrt(3)
  Demux1 : Demux  Outputs=2
  Gain1 : Gain  Gain=1/2
  Product : Product  Inputs=*/  RndMeth=Zero
  Product1 : Product  Inputs=*/  RndMeth=Zero
  Product2 : Product  Inputs=**  RndMeth=Zero
  Real-Imag to Complex : RealImagToComplex
  Trigonometric Function : Trigonometry
  Uabc_ref : Outport  VectorParamsAs1DForOutWhenUnconnected=off
  wires:
  Product/1 -> Product1/2
  Constant4/1 -> Add1/4
  wt/1 -> Add1/1
  Product2/1 -> Uabc_ref/1
  Trigonometric Function/1 -> Product2/2
  Complex to Magnitude-Angle/1 -> Product2/1
  Add2/1 -> Trigonometric Function/1
  Add1/1 -> Add2/2
  Complex to Magnitude-Angle/2 -> Add2/1
  Constant6/1 -> Product/2
  Constant/1 -> Add1/3
  Constant2/1 -> Add1/2
  Demux1/2 -> Real-Imag to Complex/2
  Demux1/1 -> Real-Imag to Complex/1
  Real-Imag to Complex/1 -> Complex to Magnitude-Angle/1
  Gain1/1 -> Product/1
  Product1/1 -> Demux1/1
  VdVq_conv/1 -> Product1/1
  Constant5/1 -> Gain1/1

== system different_inverter_controls_BPS/IBR-GFM Power Synchronization/Inverter/Inverter Control/current limiter/P priority limit ==
  idiqP : Inport
  Demux4 : Demux  Outputs=2
  IqLimit : Subsystem
  Mux4 : Mux  Inputs=2
  Rtot_pu1 : Gain  Gain=-1  SaturateOnIntegerOverflow=on  OutDataTypeStr=Inherit: Same as input  ParamDataTypeStr=Inherit: Same as input
  Saturation : Saturate  UpperLimit=limMax  LowerLimit=0
  Saturation Dynamic : simulink/Discontinuities/Saturation Dynamic  OutMin=[]  OutMax=[limMax]  OutDataTypeStr=Inherit: Same as second input  OutDataType=fixdt(1, 16)  OutScaling=2^-10  DoSatur=off
  idiqPRefL : Outport
  wires:
  Saturation Dynamic/1 -> Mux4/2
  idiqP/1 -> Demux4/1
  Demux4/2 -> Saturation Dynamic/2
  Mux4/1 -> idiqPRefL/1
  Demux4/1 -> Saturation/1
  Saturation/1 -> IqLimit/1(In1), Mux4/1
  Rtot_pu1/1 -> Saturation Dynamic/3
  IqLimit/1(Out2) -> Rtot_pu1/1, Saturation Dynamic/1

== system different_inverter_controls_BPS/IBR-GFM Power Synchronization/Inverter/Inverter Control/current limiter/Q priority limit ==
  idiqP : Inport
  V_inv_mag : Inport  Port=2
  Demux4 : Demux  Outputs=2
  Iq condition : Switch  Threshold=0.9  SaturateOnIntegerOverflow=off  InputSameDT=off
  IqLimit : Subsystem
  Mux4 : Mux  Inputs=2
  Rtot_pu1 : Gain  Gain=-1  SaturateOnIntegerOverflow=on  OutDataTypeStr=Inherit: Same as input  ParamDataTypeStr=Inherit: Same as input
  Saturation : Saturate  UpperLimit=limMax  LowerLimit=limMin
  Saturation Dynamic : simulink/Discontinuities/Saturation Dynamic  OutMin=[]  OutMax=[]  OutDataTypeStr=Inherit: Same as second input  OutDataType=fixdt(1, 16)  OutScaling=2^-10  DoSatur=off
  Saturation1 : Saturate  UpperLimit=0  LowerLimit=limMin
  Scope : Scope
  idiqPRefL : Outport
  wires:
  Iq condition/1 -> Mux4/2, IqLimit/1(In1)
  V_inv_mag/1 -> Iq condition/2
  Saturation/1 -> Iq condition/1
  idiqP/1 -> Demux4/1
  Mux4/1 -> idiqPRefL/1
  Rtot_pu1/1 -> Saturation Dynamic/3
  Saturation Dynamic/1 -> Mux4/1
  Demux4/1 -> Saturation Dynamic/2
  IqLimit/1(Out2) -> Rtot_pu1/1, Saturation Dynamic/1
  Saturation1/1 -> Iq condition/3
  Demux4/2 -> Saturation/1, Saturation1/1

== system different_inverter_controls_BPS/IBR-GFM Power Synchronization/Inverter/Inverter Control/current limiter/Subsystem3 ==
  In1 : Inport
  Demux2 : Demux  Outputs=2
  Math Function : Math  Operator=square  SignedPower=on
  Saturation : Saturate  UpperLimit=limMax  LowerLimit=limMin
  Scope : Scope  NumInputPorts=2
  Sqrt1 : Sqrt
  Subtract : Sum
  Out1 : Outport
  Out2 : Outport  Port=2
  wires:
  Demux2/2 -> Subtract/2
  Demux2/1 -> Subtract/1
  Math Function/1 -> Demux2/1
  In1/1 -> Scope/2, Math Function/1
  Subtract/1 -> Sqrt1/1  "Ipos2"
  Sqrt1/1 -> Saturation/1, Scope/1, Out2/1
  Saturation/1 -> Out1/1

== system different_inverter_controls_BPS/IBR-GFM Power Synchronization/Inverter/Inverter Control/current limiter/Subsystem4 ==
  In1 : Inport
  In2 : Inport  Port=2
  Demux4 : Demux  Outputs=2
  Mux4 : Mux  Inputs=2
  Switch1 : Switch  Threshold=limMax  SaturateOnIntegerOverflow=off  InputSameDT=off
  Unit Delay2 : UnitDelay  InitialCondition=1  SampleTime=Ts_Control  HasFrameUpgradeWarning=on
  dummy limit : Saturate  UpperLimit=limMax  LowerLimit=limMin
  Out1 : Outport
  wires:
  Switch1/1 -> Out1/1, Mux4/1, Unit Delay2/1
  Unit Delay2/1 -> Switch1/1
  In1/1 -> Switch1/2
  In2/1 -> Switch1/3, Demux4/1
  Demux4/2 -> dummy limit/1
  dummy limit/1 -> Mux4/2

== system different_inverter_controls_BPS/IBR-GFM Power Synchronization/Inverter/Inverter Control/current limiter/Subsystem9 ==
  In1 : Inport
  In2 : Inport  Port=2
  Divide : Product  Inputs=*/
  Gain1 : Gain  Gain=limMax
  Saturation : Saturate  UpperLimit=limMax  LowerLimit=limMin
  Switch1 : Switch  Threshold=limMax  SaturateOnIntegerOverflow=off  InputSameDT=off
  idiqPRefL : Outport
  wires:
  In1/1 -> Divide/2, Switch1/2
  In2/1 -> Divide/1, Switch1/3
  Divide/1 -> Gain1/1
  Gain1/1 -> Switch1/1
  Switch1/1 -> Saturation/1
  Saturation/1 -> idiqPRefL/1

== system different_inverter_controls_BPS/IBR-GFM Power Synchronization/Inverter/Power Controller/P,Q Control /Integrator ==
  w : Inport
  Constant1 : Constant  Commented=on  Value=2*pi  SampleTime=Ts
  Constant2 : Constant  Value=2*pi  SampleTime=Ts_Control
  Constant3 : Constant  Commented=on  Value=2*pi  SampleTime=Ts
  Constant4 : Constant  Commented=on  Value=f  SampleTime=Ts_Control
  Constant5 : Constant  Commented=on  Value=0  SampleTime=Ts_Control
  Discrete-Time Integrator : DiscreteIntegrator  Commented=on  IntegratorMethod=Integration: Trapezoidal  SampleTime=Ts  ICPrevOutput=DiscIntNeverNeededParam  ICPrevScaledInput=DiscIntNeverNeededParam
  Discrete-Time Integrator1 : DiscreteIntegrator  ExternalReset=rising  InitialConditionSource=external  SampleTime=Ts_Control  ShowStatePort=on  ICPrevOutput=DiscIntNeverNeededParam  ICPrevScaledInput=DiscIntNeverNeededParam
  Divide : Product  Commented=on  Inputs=*/
  From : From  Commented=on  GotoTag=fsys
  Gain : Gain  Commented=on  Gain=2*pi*f
  Gain1 : Gain  Commented=on  Gain=2*pi*f  SaturateOnIntegerOverflow=on  OutDataTypeStr=Inherit: Same as input  ParamDataTypeStr=Inherit: Same as input
  Gain3 : Gain  Gain=2*pi*f
  Hit Crossing : HitCross  Commented=on  HitCrossingOffset=pi  HitCrossingDirection=falling  ShowOutputPort=off
  Initial : InitialCondition  Value=0
  Initial1 : InitialCondition  Commented=on  Value=0
  Integrator : Integrator  Commented=on  ExternalReset=rising  InitialConditionSource=external  InitialCondition=sps.Phase_Init*pi/180  LimitOutput=on  ShowStatePort=on
  Integrator2 : Integrator  Commented=on  ExternalReset=rising  InitialConditionSource=external  InitialCondition=sps.Phase_Init*pi/180  ShowStatePort=on
  Math Function : Math  Commented=on  Operator=mod  SignedPower=on
  Relational Operator : RelationalOperator  Operator=>  OutDataTypeStr=boolean  InputSameDT=off
  Relational Operator1 : RelationalOperator  Commented=on  Operator=>  OutDataTypeStr=boolean  InputSameDT=off
  Scope : Scope
  Scope1 : Scope  Commented=on
  Scope2 : Scope  Commented=on
  Scope3 : Scope  Commented=on
  Subtract : Sum  Inputs=+-
  Subtract1 : Sum  Commented=on  Inputs=+-
  Sum1 : Sum  Commented=on  Inputs=|++
  Sum2 : Sum  Commented=on  Inputs=|+-
  Theta : Outport
  wires:
  Gain3/1 -> Discrete-Time Integrator1/1
  w/1 -> Sum2/1, Gain3/1
  Gain1/1 -> Integrator/1
  Initial1/1 -> Integrator/3
  Relational Operator1/1 -> Integrator/2
  Integrator/State -> Subtract1/1, Relational Operator1/1
  Constant1/1 -> Subtract1/2, Relational Operator1/2
  Integrator/1 -> Scope3/1, Hit Crossing/1
  Subtract1/1 -> Initial1/1
  Relational Operator/1 -> Discrete-Time Integrator1/2
  Initial/1 -> Discrete-Time Integrator1/3
  Discrete-Time Integrator1/State -> Subtract/1, Relational Operator/1
  Constant2/1 -> Subtract/2, Relational Operator/2
  Subtract/1 -> Initial/1
  Discrete-Time Integrator1/1 -> Scope/1, Theta/1
  Gain/1 -> Discrete-Time Integrator/1
  Discrete-Time Integrator/1 -> Math Function/1
  Constant3/1 -> Math Function/2
  Math Function/1 -> Scope1/1
  Sum1/1 -> Gain/1  "W"
  Constant5/1 -> Sum2/2
  Sum2/1 -> Scope2/1, Sum1/1  "W"
  From/1 -> Divide/1
  Constant4/1 -> Divide/2
  Divide/1 -> Sum1/2
